simulink model "RC_Circuit2"  (R2020a)
settings: Solver=VariableStepAuto  StartTime=0.0  StopTime=10  RelTol=1e-5
values from neighbouring files (symbols this model uses):
  C = 100e-5    (= 0.001)    [RC_Circuit_param.m]
  f = f_range(i)    [RC_Circuit_param.m]
  R = 1    [RC_Circuit_param.m]
  U = 1    [RC_Circuit_param.m]
settings Model: Creator=barni  LastModifiedBy=MBr
settings DataIOCC: Refine=100

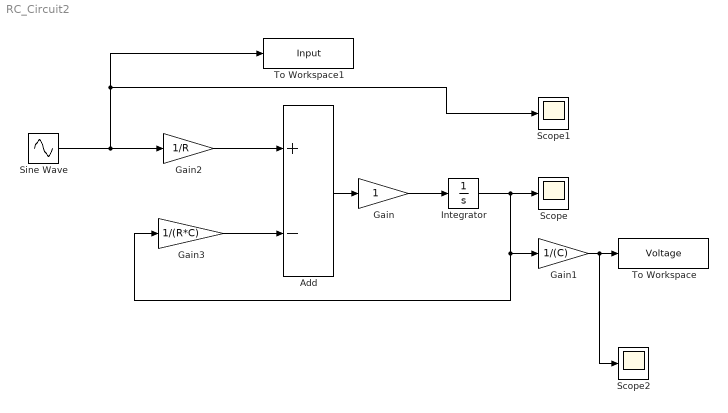
== system RC_Circuit2 ==
  Add : Sum  Inputs=+-
  Gain : Gain
  Gain1 : Gain  Gain=1/(C)
  Gain2 : Gain  Gain=1/R
  Gain3 : Gain  Gain=1/(R*C)
  Integrator : Integrator
  Scope : Scope
  Scope1 : Scope
  Scope2 : Scope
  Sine Wave : Sin  Amplitude=U  Frequency=2*pi*f  SampleTime=0
  To Workspace : ToWorkspace  VariableName=Voltage  SaveFormat=Structure With Time  SampleTime=-1
  To Workspace1 : ToWorkspace  VariableName=Input  SaveFormat=Structure With Time  SampleTime=-1
  wires:
  Sine Wave/1 -> Gain2/1, To Workspace1/1, Scope1/1
  Add/1 -> Gain/1
  Gain/1 -> Integrator/1
  Integrator/1 -> Scope/1, Gain1/1, Gain3/1
  Gain1/1 -> Scope2/1, To Workspace/1
  Gain2/1 -> Add/1
  Gain3/1 -> Add/2
